simulink model "Test4_wind_withDCconverter"  (R2022b)
settings: Solver=VariableStepAuto  StartTime=0.0  StopTime=10.0  RelTol=1e-3
libraries: fl_lib x36, ee_lib x12, nesl_utility x12, eeDcDcVoltageController x1, eePwmGenerator x1
settings Model: Creator=lenovo  LastModifiedBy=lenovo

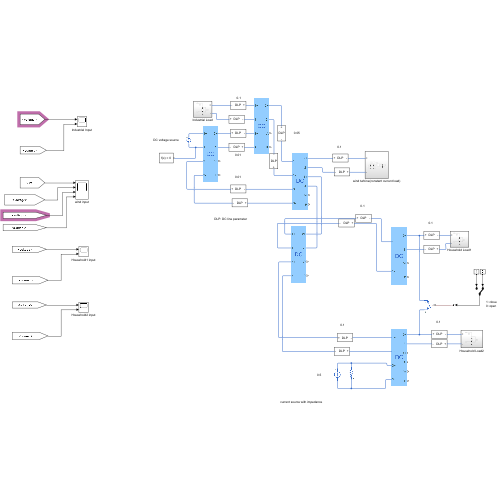
[thumbnail: Simulink's stored preview of the top-level diagram]
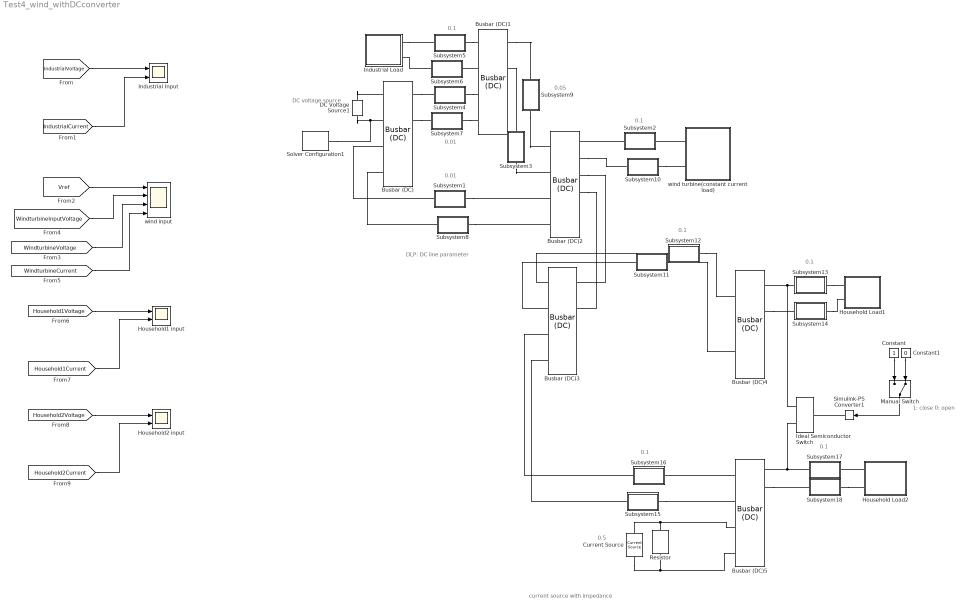
== system Test4_wind_withDCconverter ==
  note: 0.1
  note: DLP: DC line parameter
  note: 1: close
      | 0: open
  note: current source with impedance
  note: DC voltage source
  note: 0.01
  note: 0.05
  note: 0.1
  note: 0.01
  note: 0.1
  note: 0.1
  note: 0.1
  note: 0.1
  note: 0.5
  Busbar (DC) : ee_lib/Connectors & References/Busbar (DC)  n_nodes=ee.enum.connectors.busbar_number_of_connections.three  VRated=1e3 V  measurement_type=ee.enum.measurementType.instantaneous  averaging_period=1e-2 s  show_ps=ee.enum.connectors.busbar_measurement.true
      settings: InternalSimscapePortConfiguration="{\"Bottom\":[],\"Left\":[{\"id\":\"p1\",\"label\":\"1+\",\"type\":\"foundation.electrical.electrical\"},{\"id\":\"n1\",\"label\":\"1-\",\"type\":\"foundation.electrical.electrical\"},{\"id\":\"p3\",\"label\":\"3+\",\"type\":\"foundation.electrical.electrical\"},{\"id\":\"n3\",\"label\":\"3-\",\"type\":\"foundation.electrical.electrical\"}],\"Right\":[{\"id\":\"p2\",\"label\":\"2+\",\"type\":\"foundation.electrical.electrical\"},{\"id\":\"n2\",\"label\":\"2-\",\"type\":\"foundation.electrical.electrical\"},{\"id\":\"Vt_ps\",\"label\":\"Vt\",\"type\":\"output\"},{\"id\":\"P3_ps\",\"label\":\"P\",\"type\":\"output\"}],\"Top\":[]}"
  Busbar (DC)1 : ee_lib/Connectors & References/Busbar (DC)  n_nodes=ee.enum.connectors.busbar_number_of_connections.three  VRated=1e3 V  measurement_type=ee.enum.measurementType.instantaneous  averaging_period=1e-2 s  show_ps=ee.enum.connectors.busbar_measurement.true
      settings: InternalSimscapePortConfiguration="{\"Bottom\":[],\"Left\":[{\"id\":\"p1\",\"label\":\"1+\",\"type\":\"foundation.electrical.electrical\"},{\"id\":\"n1\",\"label\":\"1-\",\"type\":\"foundation.electrical.electrical\"},{\"id\":\"p3\",\"label\":\"3+\",\"type\":\"foundation.electrical.electrical\"},{\"id\":\"n3\",\"label\":\"3-\",\"type\":\"foundation.electrical.electrical\"}],\"Right\":[{\"id\":\"p2\",\"label\":\"2+\",\"type\":\"foundation.electrical.electrical\"},{\"id\":\"n2\",\"label\":\"2-\",\"type\":\"foundation.electrical.electrical\"},{\"id\":\"Vt_ps\",\"label\":\"Vt\",\"type\":\"output\"},{\"id\":\"P3_ps\",\"label\":\"P\",\"type\":\"output\"}],\"Top\":[]}"
  Busbar (DC)2 : ee_lib/Connectors & References/Busbar (DC)  n_nodes=ee.enum.connectors.busbar_number_of_connections.four  VRated=1e3 V  measurement_type=ee.enum.measurementType.instantaneous  averaging_period=1e-2 s  show_ps=ee.enum.connectors.busbar_measurement.true
      settings: InternalSimscapePortConfiguration="{\"Bottom\":[],\"Left\":[{\"id\":\"p1\",\"label\":\"1+\",\"type\":\"foundation.electrical.electrical\"},{\"id\":\"n1\",\"label\":\"1-\",\"type\":\"foundation.electrical.electrical\"},{\"id\":\"p3\",\"label\":\"3+\",\"type\":\"foundation.electrical.electrical\"},{\"id\":\"n3\",\"label\":\"3-\",\"type\":\"foundation.electrical.electrical\"}],\"Right\":[{\"id\":\"p2\",\"label\":\"2+\",\"type\":\"foundation.electrical.electrical\"},{\"id\":\"n2\",\"label\":\"2-\",\"type\":\"foundation.electrical.electrical\"},{\"id\":\"p4\",\"label\":\"4+\",\"type\":\"foundation.electrical.electrical\"},{\"id\":\"n4\",\"label\":\"4-\",\"type\":\"foundation.electrical.electrical\"},{\"id\":\"Vt_ps\",\"label\":\"Vt\",\"type\":\"output\"},{\"id\":\"P4_ps\",\"label\":\"P\",\"type\":\"output\"}],\"Top\":[]}"
  Busbar (DC)3 : ee_lib/Connectors & References/Busbar (DC)  n_nodes=ee.enum.connectors.busbar_number_of_connections.three  VRated=1e3 V  measurement_type=ee.enum.measurementType.instantaneous  averaging_period=1e-2 s  show_ps=ee.enum.connectors.busbar_measurement.true
      settings: InternalSimscapePortConfiguration="{\"Bottom\":[],\"Left\":[{\"id\":\"p1\",\"label\":\"1+\",\"type\":\"foundation.electrical.electrical\"},{\"id\":\"n1\",\"label\":\"1-\",\"type\":\"foundation.electrical.electrical\"},{\"id\":\"p3\",\"label\":\"3+\",\"type\":\"foundation.electrical.electrical\"},{\"id\":\"n3\",\"label\":\"3-\",\"type\":\"foundation.electrical.electrical\"}],\"Right\":[{\"id\":\"p2\",\"label\":\"2+\",\"type\":\"foundation.electrical.electrical\"},{\"id\":\"n2\",\"label\":\"2-\",\"type\":\"foundation.electrical.electrical\"},{\"id\":\"Vt_ps\",\"label\":\"Vt\",\"type\":\"output\"},{\"id\":\"P3_ps\",\"label\":\"P\",\"type\":\"output\"}],\"Top\":[]}"
  Busbar (DC)4 : ee_lib/Connectors & References/Busbar (DC)  n_nodes=ee.enum.connectors.busbar_number_of_connections.two  VRated=1e3 V  measurement_type=ee.enum.measurementType.instantaneous  averaging_period=1e-2 s  show_ps=ee.enum.connectors.busbar_measurement.true
      settings: InternalSimscapePortConfiguration="{\"Bottom\":[],\"Left\":[{\"id\":\"p1\",\"label\":\"1+\",\"type\":\"foundation.electrical.electrical\"},{\"id\":\"n1\",\"label\":\"1-\",\"type\":\"foundation.electrical.electrical\"}],\"Right\":[{\"id\":\"p2\",\"label\":\"2+\",\"type\":\"foundation.electrical.electrical\"},{\"id\":\"n2\",\"label\":\"2-\",\"type\":\"foundation.electrical.electrical\"},{\"id\":\"Vt_ps\",\"label\":\"Vt\",\"type\":\"output\"},{\"id\":\"P2_ps\",\"label\":\"P\",\"type\":\"output\"}],\"Top\":[]}"
  Busbar (DC)5 : ee_lib/Connectors & References/Busbar (DC)  n_nodes=ee.enum.connectors.busbar_number_of_connections.four  VRated=1e3 V  measurement_type=ee.enum.measurementType.instantaneous  averaging_period=1e-2 s  show_ps=ee.enum.connectors.busbar_measurement.true
      settings: InternalSimscapePortConfiguration="{\"Bottom\":[],\"Left\":[{\"id\":\"p1\",\"label\":\"1+\",\"type\":\"foundation.electrical.electrical\"},{\"id\":\"n1\",\"label\":\"1-\",\"type\":\"foundation.electrical.electrical\"},{\"id\":\"p3\",\"label\":\"3+\",\"type\":\"foundation.electrical.electrical\"},{\"id\":\"n3\",\"label\":\"3-\",\"type\":\"foundation.electrical.electrical\"}],\"Right\":[{\"id\":\"p2\",\"label\":\"2+\",\"type\":\"foundation.electrical.electrical\"},{\"id\":\"n2\",\"label\":\"2-\",\"type\":\"foundation.electrical.electrical\"},{\"id\":\"p4\",\"label\":\"4+\",\"type\":\"foundation.electrical.electrical\"},{\"id\":\"n4\",\"label\":\"4-\",\"type\":\"foundation.electrical.electrical\"},{\"id\":\"Vt_ps\",\"label\":\"Vt\",\"type\":\"output\"},{\"id\":\"P4_ps\",\"label\":\"P\",\"type\":\"output\"}],\"Top\":[]}"
  Constant : Constant
  Constant1 : Constant  Value=0
  Current Source : ee_lib/Sources/Current Source  dc_current=0.5 A  ac_current=0 A  ac_shift=0 rad  ac_frequency=60 Hz  noise_mode=ee.enum.sources.noise.Disabled  PSD=0 A^2/Hz  sample_time=1e-3 s  repeatability=ee.enum.sources.repeatability.NotRepeatable  user_seed=0  auto_seed=3499211588  i_specify=off  i_priority=None  i=0 A  i_nominal_specify=off  i_nominal_unit=A  i_nominal_value=1  v_specify=off  v_priority=None  v=0 V  v_nominal_specify=off  v_nominal_unit=V  v_nominal_value=1
  DC Voltage Source1 : ee_lib/Additional Components/SPICE Sources/DC Voltage Source  DC=5 V
  Household Load1 : Subsystem
  Household Load2 : Subsystem
  Household1 input : Scope  NumInputPorts=2
  Household2 input : Scope  NumInputPorts=2
  Ideal Semiconductor Switch : ee_lib/Semiconductors & Converters/Ideal Semiconductor Switch  port_option=ee.enum.controlport.ps  Ron=0.001 Ohm  Goff=1e-6 1/Ohm  Vth=0.5 V  diode_param=ee.enum.converters.protectiondiode.none  diode_Vf=0.8 V  diode_Ron=0.001 Ohm  diode_Goff=1e-5 1/Ohm  diode_C=50e-9 F  diode_iRM=-235 A  diode_iF=300 A  diode_idot=-50 A/us  diode_trr_param=ee.enum.converters.diodetrr.trr_factor  diode_trr_factor=3  diode_trr=15 us  diode_Qrr=1500 s*uA
  Industrial Input : Scope  NumInputPorts=2
  Industrial Load : Subsystem
  Manual Switch : ManualSwitch  CurrentSetting=0
  Resistor : ee_lib/Passive/Resistor  R=1 Ohm  enable_R_tol=0  R_tol=5  tol_distribution=1  nSigma=4  enable_operating_limits=0  operating_limit_action=2  max_working_voltage=100 V  power_rating=1 W  enable_faults=0  fault_action=1  R_faulted=inf Ohm  enable_temporal_fault=0  t_fault=1 s  enable_behavioral_fault=0  max_permissible_current=1 A  t_fail_on_current=1 s  noise_mode=0  sample_time=1e-3 s  repeatability=1  auto_seed=3890346746  user_seed=0  Tdevice=25 degC  power_derating_T1=70 degC  power_derating_T2=155 degC  operating_temperature_range_vec=[-50, 150] degC  alpha=3.93e-3 1/K  Tmeas=25 degC  thermal_mass=100 J/K  temperature_specify=off  temperature_priority=High  temperature=298.15 K  temperature_nominal_specify=off  temperature_nominal_unit=K  temperature_nominal_value=1
  Simulink-PS Converter1 : nesl_utility/Simulink-PS Converter  PhysicalDomain=network_engine_domain  SubClassName=ps_input  LeftPortType=input  RightPortType=output  PseudoPeriodic=off  Frequencies=[]  NoiseDistribution=none  NoiseParameters=[]  Unit=1  AffineConversion=off  FilteringAndDerivatives=provide  SimscapeFilterOrder=1  InputFilterTimeConstant=0.001  UdotUserProvided=0
  Solver Configuration1 : nesl_utility/Solver Configuration  PhysicalDomain=network_engine_domain  SubClassName=solver  LeftPortType=input  RightPortType=generic  Tones=[]  Harmonics=[]  SimulateNoise=off  Profile=off  UseLocalSampling=off  EnableSwitchedLinearOptims=on  FrequencyDomain=off  UseCCode=off  RelTol=0.001  AbsTol=1e-06  MinStep=1e-09  ToWorkspace=off  RevertToSquareIcSolve=off  NumHomotopyIterations=100  PhasorMode=off  PhasorModeNumHarmonics=1  ConsistencySolver=NEWTON_FTOL  IndexReductionMethod=DerivativeReplacement  DoDC=off  ResidualTolerance=1e-9  ConsistencyTolSource=GLOBAL  ConsistencyAbsTol=0.001  ConsistencyRelTol=0.001  ConsistencyTolFactor=0.001  UseLocalSolver=on  LocalSolverChoice=NE_BACKWARD_EULER_ADVANCER  ResolveIndetEquations=on  FunctionEvalNumThread=1  LocalSolverSampleTime=5e-6  DoFixedCost=on  MaxNonlinIter=3  MaxModeIter=2  ComputeImpulses=off  ImpulseIterations=2  LinearAlgebra=auto  LinearAlgebraNumThread=0  EquationFormulation=NE_TIME_EF  DelaysMemoryBudget=1024  AutomaticFiltering=on  FilteringTimeConstant=0.001  PartitionStorageMethod=AS_NEEDED  PartitionMemoryBudget=1024  PartitionMethod=FAST
  Subsystem1 : Subsystem
      mask Display:
      | disp('DLP')
      | port_label('LConn',1,'+')
      | port_label('RConn',1,'-')
  Subsystem10 : Subsystem
      mask Display:
      | disp('DLP')
      | port_label('LConn',1,'+')
      | port_label('RConn',1,'-')
  Subsystem11 : Subsystem
      mask Display:
      | disp('DLP')
      | port_label('LConn',1,'+')
      | port_label('RConn',1,'-')
  Subsystem12 : Subsystem
      mask Display:
      | disp('DLP')
      | port_label('LConn',1,'+')
      | port_label('RConn',1,'-')
  Subsystem13 : Subsystem
      mask Display:
      | disp('DLP')
      | port_label('LConn',1,'+')
      | port_label('RConn',1,'-')
  Subsystem14 : Subsystem
      mask Display:
      | disp('DLP')
      | port_label('LConn',1,'+')
      | port_label('RConn',1,'-')
  Subsystem15 : Subsystem
      mask Display:
      | disp('DLP')
      | port_label('LConn',1,'+')
      | port_label('RConn',1,'-')
  Subsystem16 : Subsystem
      mask Display:
      | disp('DLP')
      | port_label('LConn',1,'+')
      | port_label('RConn',1,'-')
  Subsystem17 : Subsystem
      mask Display:
      | disp('DLP')
      | port_label('LConn',1,'+')
      | port_label('RConn',1,'-')
  Subsystem18 : Subsystem
      mask Display:
      | disp('DLP')
      | port_label('LConn',1,'+')
      | port_label('RConn',1,'-')
  Subsystem2 : Subsystem
      mask Display:
      | disp('DLP')
      | port_label('LConn',1,'+')
      | port_label('RConn',1,'-')
  Subsystem3 : Subsystem
      mask Display:
      | disp('DLP')
      | port_label('LConn',1,'+')
      | port_label('RConn',1,'-')
  Subsystem4 : Subsystem
      mask Display:
      | disp('DLP')
      | port_label('LConn',1,'+')
      | port_label('RConn',1,'-')
  Subsystem5 : Subsystem
      mask Display:
      | disp('DLP')
      | port_label('LConn',1,'+')
      | port_label('RConn',1,'-')
  Subsystem6 : Subsystem
      mask Display:
      | disp('DLP')
      | port_label('LConn',1,'+')
      | port_label('RConn',1,'-')
  Subsystem7 : Subsystem
      mask Display:
      | disp('DLP')
      | port_label('LConn',1,'+')
      | port_label('RConn',1,'-')
  Subsystem8 : Subsystem
      mask Display:
      | disp('DLP')
      | port_label('LConn',1,'+')
      | port_label('RConn',1,'-')
  Subsystem9 : Subsystem
      mask Display:
      | disp('DLP')
      | port_label('LConn',1,'+')
      | port_label('RConn',1,'-')
  wind input : Scope  NumInputPorts=4
  wind turbine(constant current load) : Subsystem
  wires:
  [IndustrialVoltage] -> Industrial Input/1
  [IndustrialCurrent] -> Industrial Input/2
  [WindturbineVoltage] -> wind input/3
  [Vref] -> wind input/1
  [WindturbineInputVoltage] -> wind input/2
  [WindturbineCurrent] -> wind input/4
  Constant/1 -> Manual Switch/1
  Manual Switch/1 -> Simulink-PS Converter1/1
  Constant1/1 -> Manual Switch/2
  [Household1Current] -> Household1 input/2
  [Household1Voltage] -> Household1 input/1
  [Household2Voltage] -> Household2 input/1
  [Household2Current] -> Household2 input/2
  connections:
  Household Load2/LConn1 -- Subsystem17/RConn1
  Busbar (DC)3/LConn2 -- Subsystem11/RConn1
  Busbar (DC)1/RConn2 -- Subsystem3/RConn1
  Subsystem16/LConn1 -- Busbar (DC)3/LConn3
  Busbar (DC)2/RConn4 -- Busbar (DC)3/RConn2
  Busbar (DC)/RConn2 -- Subsystem7/RConn1
  Busbar (DC)/LConn3 -- Subsystem1/LConn1
  Subsystem15/LConn1 -- Busbar (DC)5/LConn2
  Busbar (DC)5/RConn2 -- Subsystem18/RConn1
  DC Voltage Source1/LConn1 -- Busbar (DC)/LConn1
  Busbar (DC)2/RConn3 -- Busbar (DC)3/RConn1
  Busbar (DC)/RConn1 -- Subsystem4/LConn1
  DC Voltage Source1/RConn1 -- Solver Configuration1/RConn1 -- Busbar (DC)/LConn2
  Busbar (DC)3/LConn1 -- Subsystem12/LConn1
  Busbar (DC)1/RConn1 -- Subsystem9/LConn1
  Busbar (DC)/LConn4 -- Subsystem8/RConn1
  Busbar (DC)1/LConn2 -- Subsystem6/RConn1
  Industrial Load/LConn1 -- Subsystem5/RConn1
  Busbar (DC)4/RConn1 -- Ideal Semiconductor Switch/RConn2 -- Subsystem13/LConn1
  Busbar (DC)4/RConn2 -- Subsystem14/RConn1
  wind turbine(constant current load)/LConn1 -- Subsystem2/RConn1
  Busbar (DC)2/RConn2 -- Subsystem10/RConn1
  Simulink-PS Converter1/RConn1 -- Ideal Semiconductor Switch/LConn1
  Current Source/LConn1 -- Resistor/LConn1 -- Busbar (DC)5/LConn3
  Current Source/RConn1 -- Resistor/RConn1 -- Busbar (DC)5/LConn4
  Subsystem1/RConn1 -- Busbar (DC)2/LConn3
  Subsystem4/RConn1 -- Busbar (DC)1/LConn3
  Subsystem5/LConn1 -- Busbar (DC)1/LConn1
  Subsystem6/LConn1 -- Industrial Load/LConn2
  Subsystem7/LConn1 -- Busbar (DC)1/LConn4
  Subsystem8/LConn1 -- Busbar (DC)2/LConn4
  Subsystem2/LConn1 -- Busbar (DC)2/RConn1
  Subsystem10/LConn1 -- wind turbine(constant current load)/LConn2
  Subsystem9/RConn1 -- Busbar (DC)2/LConn1
  Subsystem3/LConn1 -- Busbar (DC)2/LConn2
  Subsystem11/LConn1 -- Busbar (DC)4/LConn2
  Subsystem12/RConn1 -- Busbar (DC)4/LConn1
  Subsystem13/RConn1 -- Household Load1/LConn1
  Subsystem14/LConn1 -- Household Load1/LConn2
  Busbar (DC)5/LConn1 -- Subsystem16/RConn1
  Subsystem15/RConn1 -- Busbar (DC)3/LConn4
  Subsystem17/LConn1 -- Busbar (DC)5/RConn1 -- Ideal Semiconductor Switch/RConn1
  Subsystem18/LConn1 -- Household Load2/LConn2

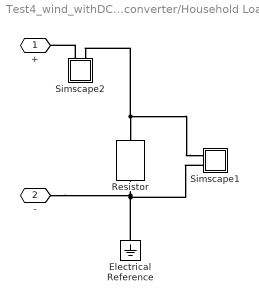
== system Test4_wind_withDCconverter/Household Load1 ==
  Electrical Reference : fl_lib/Electrical/Electrical Elements/Electrical Reference
  Resistor : fl_lib/Electrical/Electrical Elements/Resistor  R=1 Ohm  i_specify=off  i_priority=None  i=0 A  i_nominal_specify=off  i_nominal_unit=A  i_nominal_value=1  v_specify=off  v_priority=None  v=0 V  v_nominal_specify=off  v_nominal_unit=V  v_nominal_value=1
  Simscape1 : Subsystem
      mask Display:
      | disp('V')
      | port_label('LConn',1,'+')
      | port_label('LConn',2,'-')
  Simscape2 : Subsystem
      mask Display:
      | disp('A')
      | port_label('LConn',1,'+')
      | port_label('LConn',2,'-')
  + : PMIOPort  Side=Left
  - : PMIOPort  Port=2  Side=Left
  connections:
  Simscape2/LConn1 -- +/RConn1
  Simscape1/LConn1 -- Simscape2/LConn2 -- Resistor/LConn1
  Simscape1/LConn2 -- Resistor/RConn1 -- -/RConn1 -- Electrical Reference/LConn1

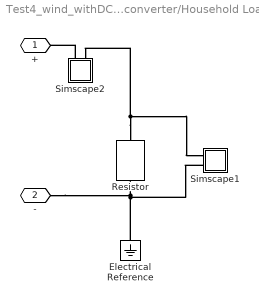
== system Test4_wind_withDCconverter/Household Load2 ==
  Electrical Reference : fl_lib/Electrical/Electrical Elements/Electrical Reference
  Resistor : fl_lib/Electrical/Electrical Elements/Resistor  R=1 Ohm  i_specify=off  i_priority=None  i=0 A  i_nominal_specify=off  i_nominal_unit=A  i_nominal_value=1  v_specify=off  v_priority=None  v=0 V  v_nominal_specify=off  v_nominal_unit=V  v_nominal_value=1
  Simscape1 : Subsystem
      mask Display:
      | disp('V')
      | port_label('LConn',1,'+')
      | port_label('LConn',2,'-')
  Simscape2 : Subsystem
      mask Display:
      | disp('A')
      | port_label('LConn',1,'+')
      | port_label('LConn',2,'-')
  + : PMIOPort  Side=Left
  - : PMIOPort  Port=2  Side=Left
  connections:
  Electrical Reference/LConn1 -- -/RConn1 -- Resistor/RConn1 -- Simscape1/LConn2
  Resistor/LConn1 -- Simscape2/LConn2 -- Simscape1/LConn1
  Simscape2/LConn1 -- +/RConn1

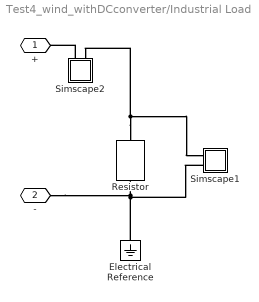
== system Test4_wind_withDCconverter/Industrial Load ==
  Electrical Reference : fl_lib/Electrical/Electrical Elements/Electrical Reference
  Resistor : fl_lib/Electrical/Electrical Elements/Resistor  R=1 Ohm  i_specify=off  i_priority=None  i=0 A  i_nominal_specify=off  i_nominal_unit=A  i_nominal_value=1  v_specify=off  v_priority=None  v=0 V  v_nominal_specify=off  v_nominal_unit=V  v_nominal_value=1
  Simscape1 : Subsystem
      mask Display:
      | disp('V')
      | port_label('LConn',1,'+')
      | port_label('LConn',2,'-')
  Simscape2 : Subsystem
      mask Display:
      | disp('A')
      | port_label('LConn',1,'+')
      | port_label('LConn',2,'-')
  + : PMIOPort  Side=Left
  - : PMIOPort  Port=2  Side=Left
  connections:
  Electrical Reference/LConn1 -- -/RConn1 -- Resistor/RConn1 -- Simscape1/LConn2
  Resistor/LConn1 -- Simscape2/LConn2 -- Simscape1/LConn1
  Simscape2/LConn1 -- +/RConn1

== system Test4_wind_withDCconverter/Subsystem1 ==
  Resistor1 : fl_lib/Electrical/Electrical Elements/Resistor  R=0.01 Ohm  i_specify=off  i_priority=None  i=0 A  i_nominal_specify=off  i_nominal_unit=A  i_nominal_value=1  v_specify=off  v_priority=None  v=0 V  v_nominal_specify=off  v_nominal_unit=V  v_nominal_value=1
  Conn1 : PMIOPort  Side=Left
  Conn2 : PMIOPort  Port=2  Side=Right
  connections:
  Resistor1/LConn1 -- Conn1/RConn1
  Resistor1/RConn1 -- Conn2/RConn1

== system Test4_wind_withDCconverter/Subsystem10 ==
  Resistor1 : fl_lib/Electrical/Electrical Elements/Resistor  R=0.1 Ohm  i_specify=off  i_priority=None  i=0 A  i_nominal_specify=off  i_nominal_unit=A  i_nominal_value=1  v_specify=off  v_priority=None  v=0 V  v_nominal_specify=off  v_nominal_unit=V  v_nominal_value=1
  Conn1 : PMIOPort  Side=Left
  Conn2 : PMIOPort  Port=2  Side=Right
  connections:
  Resistor1/RConn1 -- Conn2/RConn1
  Resistor1/LConn1 -- Conn1/RConn1

== system Test4_wind_withDCconverter/Subsystem11 ==
  Resistor1 : fl_lib/Electrical/Electrical Elements/Resistor  R=0.1 Ohm  i_specify=off  i_priority=None  i=0 A  i_nominal_specify=off  i_nominal_unit=A  i_nominal_value=1  v_specify=off  v_priority=None  v=0 V  v_nominal_specify=off  v_nominal_unit=V  v_nominal_value=1
  Conn1 : PMIOPort  Side=Left
  Conn2 : PMIOPort  Port=2  Side=Right
  connections:
  Resistor1/LConn1 -- Conn1/RConn1
  Resistor1/RConn1 -- Conn2/RConn1

== system Test4_wind_withDCconverter/Subsystem12 ==
  Resistor1 : fl_lib/Electrical/Electrical Elements/Resistor  R=0.1 Ohm  i_specify=off  i_priority=None  i=0 A  i_nominal_specify=off  i_nominal_unit=A  i_nominal_value=1  v_specify=off  v_priority=None  v=0 V  v_nominal_specify=off  v_nominal_unit=V  v_nominal_value=1
  Conn1 : PMIOPort  Side=Left
  Conn2 : PMIOPort  Port=2  Side=Right
  connections:
  Resistor1/RConn1 -- Conn2/RConn1
  Resistor1/LConn1 -- Conn1/RConn1

== system Test4_wind_withDCconverter/Subsystem13 ==
  Resistor1 : fl_lib/Electrical/Electrical Elements/Resistor  R=0.1 Ohm  i_specify=off  i_priority=None  i=0 A  i_nominal_specify=off  i_nominal_unit=A  i_nominal_value=1  v_specify=off  v_priority=None  v=0 V  v_nominal_specify=off  v_nominal_unit=V  v_nominal_value=1
  Conn1 : PMIOPort  Side=Left
  Conn2 : PMIOPort  Port=2  Side=Right
  connections:
  Resistor1/LConn1 -- Conn1/RConn1
  Resistor1/RConn1 -- Conn2/RConn1

== system Test4_wind_withDCconverter/Subsystem14 ==
  Resistor1 : fl_lib/Electrical/Electrical Elements/Resistor  R=0.1 Ohm  i_specify=off  i_priority=None  i=0 A  i_nominal_specify=off  i_nominal_unit=A  i_nominal_value=1  v_specify=off  v_priority=None  v=0 V  v_nominal_specify=off  v_nominal_unit=V  v_nominal_value=1
  Conn1 : PMIOPort  Side=Left
  Conn2 : PMIOPort  Port=2  Side=Right
  connections:
  Resistor1/RConn1 -- Conn2/RConn1
  Resistor1/LConn1 -- Conn1/RConn1

== system Test4_wind_withDCconverter/Subsystem15 ==
  Resistor1 : fl_lib/Electrical/Electrical Elements/Resistor  R=0.1 Ohm  i_specify=off  i_priority=None  i=0 A  i_nominal_specify=off  i_nominal_unit=A  i_nominal_value=1  v_specify=off  v_priority=None  v=0 V  v_nominal_specify=off  v_nominal_unit=V  v_nominal_value=1
  Conn1 : PMIOPort  Side=Left
  Conn2 : PMIOPort  Port=2  Side=Right
  connections:
  Resistor1/RConn1 -- Conn2/RConn1
  Resistor1/LConn1 -- Conn1/RConn1

== system Test4_wind_withDCconverter/Subsystem16 ==
  Resistor1 : fl_lib/Electrical/Electrical Elements/Resistor  R=0.1 Ohm  i_specify=off  i_priority=None  i=0 A  i_nominal_specify=off  i_nominal_unit=A  i_nominal_value=1  v_specify=off  v_priority=None  v=0 V  v_nominal_specify=off  v_nominal_unit=V  v_nominal_value=1
  Conn1 : PMIOPort  Side=Left
  Conn2 : PMIOPort  Port=2  Side=Right
  connections:
  Resistor1/LConn1 -- Conn1/RConn1
  Resistor1/RConn1 -- Conn2/RConn1

== system Test4_wind_withDCconverter/Subsystem17 ==
  Resistor1 : fl_lib/Electrical/Electrical Elements/Resistor  R=0.1 Ohm  i_specify=off  i_priority=None  i=0 A  i_nominal_specify=off  i_nominal_unit=A  i_nominal_value=1  v_specify=off  v_priority=None  v=0 V  v_nominal_specify=off  v_nominal_unit=V  v_nominal_value=1
  Conn1 : PMIOPort  Side=Left
  Conn2 : PMIOPort  Port=2  Side=Right
  connections:
  Resistor1/RConn1 -- Conn2/RConn1
  Resistor1/LConn1 -- Conn1/RConn1

== system Test4_wind_withDCconverter/Subsystem18 ==
  Resistor1 : fl_lib/Electrical/Electrical Elements/Resistor  R=0.1 Ohm  i_specify=off  i_priority=None  i=0 A  i_nominal_specify=off  i_nominal_unit=A  i_nominal_value=1  v_specify=off  v_priority=None  v=0 V  v_nominal_specify=off  v_nominal_unit=V  v_nominal_value=1
  Conn1 : PMIOPort  Side=Left
  Conn2 : PMIOPort  Port=2  Side=Right
  connections:
  Resistor1/LConn1 -- Conn1/RConn1
  Resistor1/RConn1 -- Conn2/RConn1

== system Test4_wind_withDCconverter/Subsystem2 ==
  Resistor1 : fl_lib/Electrical/Electrical Elements/Resistor  R=0.1 Ohm  i_specify=off  i_priority=None  i=0 A  i_nominal_specify=off  i_nominal_unit=A  i_nominal_value=1  v_specify=off  v_priority=None  v=0 V  v_nominal_specify=off  v_nominal_unit=V  v_nominal_value=1
  Conn1 : PMIOPort  Side=Left
  Conn2 : PMIOPort  Port=2  Side=Right
  connections:
  Resistor1/RConn1 -- Conn2/RConn1
  Resistor1/LConn1 -- Conn1/RConn1

== system Test4_wind_withDCconverter/Subsystem3 ==
  Resistor1 : fl_lib/Electrical/Electrical Elements/Resistor  R=0.05 Ohm  i_specify=off  i_priority=None  i=0 A  i_nominal_specify=off  i_nominal_unit=A  i_nominal_value=1  v_specify=off  v_priority=None  v=0 V  v_nominal_specify=off  v_nominal_unit=V  v_nominal_value=1
  Conn1 : PMIOPort  Side=Left
  Conn2 : PMIOPort  Port=2  Side=Right
  connections:
  Resistor1/LConn1 -- Conn1/RConn1
  Resistor1/RConn1 -- Conn2/RConn1

== system Test4_wind_withDCconverter/Subsystem4 ==
  Resistor1 : fl_lib/Electrical/Electrical Elements/Resistor  R=0.01 Ohm  i_specify=off  i_priority=None  i=0 A  i_nominal_specify=off  i_nominal_unit=A  i_nominal_value=1  v_specify=off  v_priority=None  v=0 V  v_nominal_specify=off  v_nominal_unit=V  v_nominal_value=1
  Conn1 : PMIOPort  Side=Left
  Conn2 : PMIOPort  Port=2  Side=Right
  connections:
  Resistor1/LConn1 -- Conn1/RConn1
  Resistor1/RConn1 -- Conn2/RConn1

== system Test4_wind_withDCconverter/Subsystem5 ==
  Resistor1 : fl_lib/Electrical/Electrical Elements/Resistor  R=0.1 Ohm  i_specify=off  i_priority=None  i=0 A  i_nominal_specify=off  i_nominal_unit=A  i_nominal_value=1  v_specify=off  v_priority=None  v=0 V  v_nominal_specify=off  v_nominal_unit=V  v_nominal_value=1
  Conn1 : PMIOPort  Side=Left
  Conn2 : PMIOPort  Port=2  Side=Right
  connections:
  Resistor1/RConn1 -- Conn2/RConn1
  Resistor1/LConn1 -- Conn1/RConn1

== system Test4_wind_withDCconverter/Subsystem6 ==
  Resistor1 : fl_lib/Electrical/Electrical Elements/Resistor  R=0.1 Ohm  i_specify=off  i_priority=None  i=0 A  i_nominal_specify=off  i_nominal_unit=A  i_nominal_value=1  v_specify=off  v_priority=None  v=0 V  v_nominal_specify=off  v_nominal_unit=V  v_nominal_value=1
  Conn1 : PMIOPort  Side=Left
  Conn2 : PMIOPort  Port=2  Side=Right
  connections:
  Resistor1/LConn1 -- Conn1/RConn1
  Resistor1/RConn1 -- Conn2/RConn1

== system Test4_wind_withDCconverter/Subsystem7 ==
  Resistor1 : fl_lib/Electrical/Electrical Elements/Resistor  R=0.01 Ohm  i_specify=off  i_priority=None  i=0 A  i_nominal_specify=off  i_nominal_unit=A  i_nominal_value=1  v_specify=off  v_priority=None  v=0 V  v_nominal_specify=off  v_nominal_unit=V  v_nominal_value=1
  Conn1 : PMIOPort  Side=Left
  Conn2 : PMIOPort  Port=2  Side=Right
  connections:
  Resistor1/RConn1 -- Conn2/RConn1
  Resistor1/LConn1 -- Conn1/RConn1

== system Test4_wind_withDCconverter/Subsystem8 ==
  Resistor1 : fl_lib/Electrical/Electrical Elements/Resistor  R=0.01 Ohm  i_specify=off  i_priority=None  i=0 A  i_nominal_specify=off  i_nominal_unit=A  i_nominal_value=1  v_specify=off  v_priority=None  v=0 V  v_nominal_specify=off  v_nominal_unit=V  v_nominal_value=1
  Conn1 : PMIOPort  Side=Left
  Conn2 : PMIOPort  Port=2  Side=Right
  connections:
  Resistor1/RConn1 -- Conn2/RConn1
  Resistor1/LConn1 -- Conn1/RConn1

== system Test4_wind_withDCconverter/Subsystem9 ==
  Resistor1 : fl_lib/Electrical/Electrical Elements/Resistor  R=0.05 Ohm  i_specify=off  i_priority=None  i=0 A  i_nominal_specify=off  i_nominal_unit=A  i_nominal_value=1  v_specify=off  v_priority=None  v=0 V  v_nominal_specify=off  v_nominal_unit=V  v_nominal_value=1
  Conn1 : PMIOPort  Side=Left
  Conn2 : PMIOPort  Port=2  Side=Right
  connections:
  Resistor1/LConn1 -- Conn1/RConn1
  Resistor1/RConn1 -- Conn2/RConn1

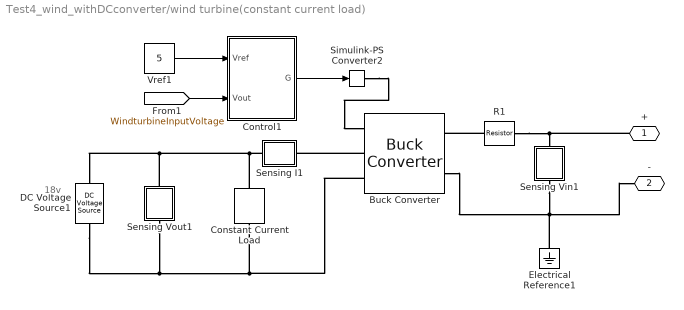
== system Test4_wind_withDCconverter/wind turbine(constant current load) ==
  note: 18v
  Buck Converter : ee_lib/Semiconductors & Converters/Converters/Buck Converter  port_option=ee.enum.controlport.ps  device_type=ee.enum.converters.switchingdevice.igbt  Vf=0.8 V  Ron=0.001 Ohm  Rds=0.001 Ohm  Goff=1e-5 1/Ohm  Vgt=1 V  Vgt_off=-1 V  Ih=1 A  Vth=3 V  K=0  diode_param=ee.enum.converters.protectiondiode.nodynamics  diode_Vf=0.8 V  diode_Ron=0.001 Ohm  diode_Goff=1e-5 1/Ohm  diode_C=50 nF  diode_iRM=-235 A  diode_iF=300 A  diode_idot=-50 A/us  diode_trr_param=ee.enum.converters.diodetrr.trr_factor  diode_trr_factor=3  diode_trr=15 us  diode_Qrr=1500 s*uA  Lf=0.0037 H  Rl=0 Ohm  Cf=1e-5 F  Rf=0.01 Ohm  snubber_type=ee.enum.converters.snubber.exclude  Cs=1e-7 F  Rs=0.1 Ohm  iL_specify=off  iL_priority=High  iL=0 A  iL_nominal_specify=off  iL_nominal_unit=A  iL_nominal_value=1  vc_specify=off  vc_priority=High  vc=0 V  vc_nominal_specify=off  vc_nominal_unit=V  vc_nominal_value=1
      settings: InternalSimscapePortConfiguration="{\"Bottom\":[],\"Left\":[{\"id\":\"G\",\"label\":\"G\",\"type\":\"input\"},{\"id\":\"p1\",\"label\":\"1+\",\"type\":\"foundation.electrical.electrical\"},{\"id\":\"n1\",\"label\":\"1-\",\"type\":\"foundation.electrical.electrical\"}],\"Right\":[{\"id\":\"p2\",\"label\":\"2+\",\"type\":\"foundation.electrical.electrical\"},{\"id\":\"n2\",\"label\":\"2-\",\"type\":\"foundation.electrical.electrical\"}],\"Top\":[]}"
  "Constant Current Load " : ee_lib/Passive/Constant Current Load  load_type=ee.enum.dc_ac.dc  consumed_current=6 A  min_supply_voltage=5 V  G_reverse=1e-6 S  deltaV=1e-3 V  consumed_current_rms=100 A  f0=60 Hz  Vrms_min=200 V  enable_fault=simscape.enum.onoff.off  open_conductance=1e-4 S  fault_action=simscape.enum.assert.action.none  fault_trigger=ee.enum.faults.faultTrigger.temporal  t_fault=1 s  max_permissible_power=inf W  t_fail_on_power=1 s  faulted_open_circuit_specify=off  faulted_open_circuit_priority=None  faulted_open_circuit=0
      settings: InternalSimscapePortConfiguration="{\"Bottom\":[],\"Left\":[{\"id\":\"p\",\"label\":\"+\",\"type\":\"foundation.electrical.electrical\"}],\"Right\":[{\"id\":\"n\",\"label\":\"-\",\"type\":\"foundation.electrical.electrical\"}],\"Top\":[]}"
  Control1 : Subsystem
  DC Voltage Source1 : fl_lib/Electrical/Electrical Sources/DC Voltage Source  v0=18 V
  Electrical Reference1 : fl_lib/Electrical/Electrical Elements/Electrical Reference
  R1 : fl_lib/Electrical/Electrical Elements/Resistor  R=0.07 Ohm  i_specify=off  i_priority=None  i=0 A  i_nominal_specify=off  i_nominal_unit=A  i_nominal_value=1  v_specify=off  v_priority=None  v=0 V  v_nominal_specify=off  v_nominal_unit=V  v_nominal_value=1
  Sensing Vin1 : Subsystem
      mask Display:
      | disp('V')
      | port_label('Lconn',1,'+')
      | port_label('Rconn',1,'-')
  Sensing Vout1 : Subsystem
      mask Display:
      | disp('V')
      | port_label('Lconn',1,'+')
      | port_label('Rconn',1,'-')
  Sensing I1 : Subsystem
      mask Display:
      | disp('I')
      | port_label('Lconn',1,'+')
      | port_label('Rconn',1,'-')
  Simulink-PS Converter2 : nesl_utility/Simulink-PS Converter  PhysicalDomain=network_engine_domain  SubClassName=ps_input  LeftPortType=input  RightPortType=output  PseudoPeriodic=off  Frequencies=[]  NoiseDistribution=none  NoiseParameters=[]  Unit=1  AffineConversion=off  FilteringAndDerivatives=provide  SimscapeFilterOrder=1  InputFilterTimeConstant=0.001  UdotUserProvided=0
  Vref1 : Constant  Value=5  SampleTime=5e-6
  + : PMIOPort  Side=Left
  - : PMIOPort  Port=2  Side=Left
  wires:
  Control1/1(G) -> Simulink-PS Converter2/1
  Vref1/1 -> Control1/1(Vref)
  [WindturbineInputVoltage] -> Control1/2(Vout)
  connections:
  Buck Converter/LConn2 -- Sensing I1/RConn1
  Sensing I1/LConn1 -- "Constant Current Load "/LConn1 -- DC Voltage Source1/LConn1 -- Sensing Vout1/LConn1
  DC Voltage Source1/RConn1 -- Sensing Vout1/RConn1 -- Buck Converter/LConn3 -- "Constant Current Load "/RConn1
  R1/RConn1 -- Buck Converter/RConn1
  R1/LConn1 -- +/RConn1 -- Sensing Vin1/LConn1
  Buck Converter/RConn2 -- Electrical Reference1/LConn1 -- -/RConn1 -- Sensing Vin1/RConn1
  Simulink-PS Converter2/RConn1 -- Buck Converter/LConn1

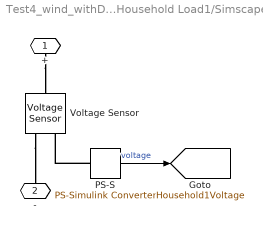
== system Test4_wind_withDCconverter/Household Load1/Simscape1 ==
  PS-S : nesl_utility/PS-Simulink Converter  PhysicalDomain=network_engine_domain  SubClassName=ps_output  LeftPortType=input  RightPortType=output  PseudoPeriodic=off  Frequencies=[]  VectorFormat=1-D array  Unit=V  AffineConversion=off
  Voltage Sensor : fl_lib/Electrical/Electrical Sensors/Voltage Sensor
  + : PMIOPort  Side=Left
  - : PMIOPort  Port=2  Side=Left
  tag scope: Household1Voltage=global
  wires:
  PS-S/1 -> [Household1Voltage]  "voltage"
  connections:
  PS-S/LConn1 -- Voltage Sensor/RConn1
  +/RConn1 -- Voltage Sensor/LConn1
  Voltage Sensor/RConn2 -- -/RConn1

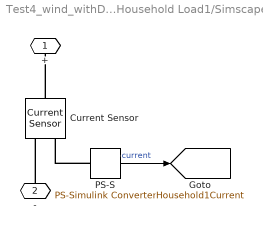
== system Test4_wind_withDCconverter/Household Load1/Simscape2 ==
  Current Sensor : fl_lib/Electrical/Electrical Sensors/Current Sensor
  PS-S : nesl_utility/PS-Simulink Converter  PhysicalDomain=network_engine_domain  SubClassName=ps_output  LeftPortType=input  RightPortType=output  PseudoPeriodic=off  Frequencies=[]  VectorFormat=1-D array  Unit=A  AffineConversion=off
  + : PMIOPort  Side=Left
  - : PMIOPort  Port=2  Side=Left
  tag scope: Household1Current=global
  wires:
  PS-S/1 -> [Household1Current]  "current"
  connections:
  -/RConn1 -- Current Sensor/RConn2
  Current Sensor/LConn1 -- +/RConn1
  PS-S/LConn1 -- Current Sensor/RConn1

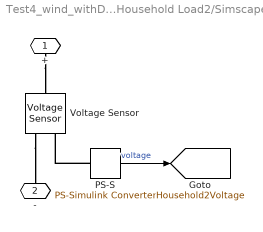
== system Test4_wind_withDCconverter/Household Load2/Simscape1 ==
  PS-S : nesl_utility/PS-Simulink Converter  PhysicalDomain=network_engine_domain  SubClassName=ps_output  LeftPortType=input  RightPortType=output  PseudoPeriodic=off  Frequencies=[]  VectorFormat=1-D array  Unit=V  AffineConversion=off
  Voltage Sensor : fl_lib/Electrical/Electrical Sensors/Voltage Sensor
  + : PMIOPort  Side=Left
  - : PMIOPort  Port=2  Side=Left
  tag scope: Household2Voltage=global
  wires:
  PS-S/1 -> [Household2Voltage]  "voltage"
  connections:
  Voltage Sensor/RConn2 -- -/RConn1
  +/RConn1 -- Voltage Sensor/LConn1
  PS-S/LConn1 -- Voltage Sensor/RConn1

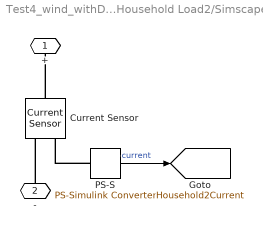
== system Test4_wind_withDCconverter/Household Load2/Simscape2 ==
  Current Sensor : fl_lib/Electrical/Electrical Sensors/Current Sensor
  PS-S : nesl_utility/PS-Simulink Converter  PhysicalDomain=network_engine_domain  SubClassName=ps_output  LeftPortType=input  RightPortType=output  PseudoPeriodic=off  Frequencies=[]  VectorFormat=1-D array  Unit=A  AffineConversion=off
  + : PMIOPort  Side=Left
  - : PMIOPort  Port=2  Side=Left
  tag scope: Household2Current=global
  wires:
  PS-S/1 -> [Household2Current]  "current"
  connections:
  PS-S/LConn1 -- Current Sensor/RConn1
  Current Sensor/LConn1 -- +/RConn1
  -/RConn1 -- Current Sensor/RConn2

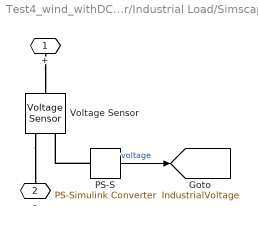
== system Test4_wind_withDCconverter/Industrial Load/Simscape1 ==
  PS-S : nesl_utility/PS-Simulink Converter  PhysicalDomain=network_engine_domain  SubClassName=ps_output  LeftPortType=input  RightPortType=output  PseudoPeriodic=off  Frequencies=[]  VectorFormat=1-D array  Unit=V  AffineConversion=off
  Voltage Sensor : fl_lib/Electrical/Electrical Sensors/Voltage Sensor
  + : PMIOPort  Side=Left
  - : PMIOPort  Port=2  Side=Left
  tag scope: IndustrialVoltage=global
  wires:
  PS-S/1 -> [IndustrialVoltage]  "voltage"
  connections:
  Voltage Sensor/RConn2 -- -/RConn1
  +/RConn1 -- Voltage Sensor/LConn1
  PS-S/LConn1 -- Voltage Sensor/RConn1

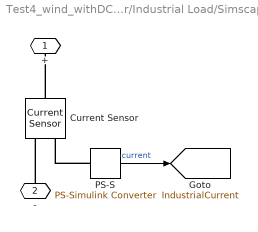
== system Test4_wind_withDCconverter/Industrial Load/Simscape2 ==
  Current Sensor : fl_lib/Electrical/Electrical Sensors/Current Sensor
  PS-S : nesl_utility/PS-Simulink Converter  PhysicalDomain=network_engine_domain  SubClassName=ps_output  LeftPortType=input  RightPortType=output  PseudoPeriodic=off  Frequencies=[]  VectorFormat=1-D array  Unit=A  AffineConversion=off
  + : PMIOPort  Side=Left
  - : PMIOPort  Port=2  Side=Left
  tag scope: IndustrialCurrent=global
  wires:
  PS-S/1 -> [IndustrialCurrent]  "current"
  connections:
  PS-S/LConn1 -- Current Sensor/RConn1
  Current Sensor/LConn1 -- +/RConn1
  -/RConn1 -- Current Sensor/RConn2

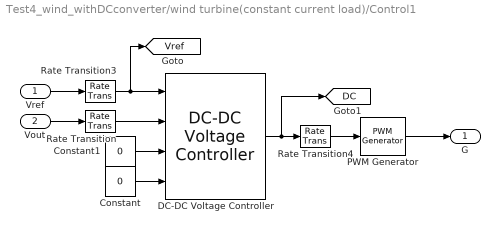
== system Test4_wind_withDCconverter/wind turbine(constant current load)/Control1 ==
  Vref : Inport
  Vout : Inport  Port=2
  Constant : Constant  Value=0
  Constant1 : Constant  Value=0
  DC-DC Voltage Controller : eeDcDcVoltageController/DC-DC Voltage Controller  Kp=0.22  Ki=46  Kaw=1  up=0.95  lo=0  Ts=1e-4  Tf=0.001  ActVdcFilter=off
  PWM Generator : eePwmGenerator/PWM Generator  CarrCount=Up  Tper=1e-4  Tdelay=0  Ts=5e-6
  Rate Transition : RateTransition  OutPortSampleTime=Tsc
  Rate Transition3 : RateTransition  OutPortSampleTime=Tsc
  Rate Transition4 : RateTransition  OutPortSampleTime=Ts
  G : Outport  VectorParamsAs1DForOutWhenUnconnected=off
  tag scope: DC=global, Vref=global
  wires:
  Rate Transition/1 -> DC-DC Voltage Controller/2
  Constant/1 -> DC-DC Voltage Controller/4
  Constant1/1 -> DC-DC Voltage Controller/3
  Rate Transition4/1 -> PWM Generator/1
  DC-DC Voltage Controller/1 -> [DC], Rate Transition4/1
  PWM Generator/1 -> G/1
  Vout/1 -> Rate Transition/1
  Rate Transition3/1 -> DC-DC Voltage Controller/1, [Vref]
  Vref/1 -> Rate Transition3/1

== system Test4_wind_withDCconverter/wind turbine(constant current load)/Sensing Vin1 ==
  PS-Simulink Converter4 : nesl_utility/PS-Simulink Converter  PhysicalDomain=network_engine_domain  SubClassName=ps_output  LeftPortType=input  RightPortType=output  PseudoPeriodic=off  Frequencies=[]  VectorFormat=1-D array  Unit=V  AffineConversion=off
  Voltage Sensor : fl_lib/Electrical/Electrical Sensors/Voltage Sensor
  + : PMIOPort  Side=Left
  - : PMIOPort  Port=2  Side=Right
  tag scope: WindturbineInputVoltage=global
  wires:
  PS-Simulink Converter4/1 -> [WindturbineInputVoltage]  "Voltage"
  connections:
  PS-Simulink Converter4/LConn1 -- Voltage Sensor/RConn1
  Voltage Sensor/RConn2 -- -/RConn1
  Voltage Sensor/LConn1 -- +/RConn1

== system Test4_wind_withDCconverter/wind turbine(constant current load)/Sensing Vout1 ==
  PS-Simulink Converter4 : nesl_utility/PS-Simulink Converter  PhysicalDomain=network_engine_domain  SubClassName=ps_output  LeftPortType=input  RightPortType=output  PseudoPeriodic=off  Frequencies=[]  VectorFormat=1-D array  Unit=V  AffineConversion=off
  Voltage Sensor : fl_lib/Electrical/Electrical Sensors/Voltage Sensor
  + : PMIOPort  Side=Left
  - : PMIOPort  Port=2  Side=Right
  tag scope: WindturbineVoltage=global
  wires:
  PS-Simulink Converter4/1 -> [WindturbineVoltage]  "voltage"
  connections:
  PS-Simulink Converter4/LConn1 -- Voltage Sensor/RConn1
  Voltage Sensor/RConn2 -- -/RConn1
  Voltage Sensor/LConn1 -- +/RConn1

== system Test4_wind_withDCconverter/wind turbine(constant current load)/Sensing I1 ==
  Current Sensor : fl_lib/Electrical/Electrical Sensors/Current Sensor
  PS-Simulink Converter3 : nesl_utility/PS-Simulink Converter  PhysicalDomain=network_engine_domain  SubClassName=ps_output  LeftPortType=input  RightPortType=output  PseudoPeriodic=off  Frequencies=[]  VectorFormat=1-D array  Unit=A  AffineConversion=off
  + : PMIOPort  Side=Left
  - : PMIOPort  Port=2  Side=Right
  tag scope: WindturbineCurrent=global
  wires:
  PS-Simulink Converter3/1 -> [WindturbineCurrent]  "Current"
  connections:
  Current Sensor/RConn1 -- PS-Simulink Converter3/LConn1
  Current Sensor/LConn1 -- +/RConn1
  Current Sensor/RConn2 -- -/RConn1
